simulink model "tank_flow"  (R2018b)
settings: Solver=ode1  StartTime=0.0  StopTime=170  FixedStep=.5  RelTol=1e-3  AbsTol=1e-6
PreLoadFcn:
  | sldemo_tankgui
StartFcn:
  | sldemo_tankgui start
StopFcn:
  | sldemo_tankgui stop
values from neighbouring files (symbols this model uses):
  Kp = 4/ts/b_lin    [tank_valve_PI_design.m]
undefined symbols (not defined in the file or in its folder): area, hilim, inflow, lolim, outflow
CloseFcn:
  | sldemo_tankgui done
Description:
  | Tank Fill and Empty with Animation
  | 
  | This example shows how to model the dynamics of liquid in a tank. The
  | associated animation provides a graphical display of the tank as it empties and
  | refills, based on user-defined tank parameters. The tank empties at the start
  | of the simulation and again part way through the simulation. When the simulation
  | is stopped, a plot is generated showing the liquid height and the states of the
  | two valves.
settings Model: ExtModeTrigMode=oneshot  ExtModeArmWhenConnect=off  ExtModeAutoUpdateStatusClock=off  Creator=The MathWorks, Inc.  LastModifiedBy=kjartan
settings SolverCC: AutoScaleAbsTol=off
settings DataIOCC: SaveFormat=Array  SignalLoggingName=sigsOut
settings OptimizationCC: InitFltsAndDblsToZero=on  LifeSpan=inf  BufferReusableBoundary=off
settings DebuggingCC: SaveWithParameterizedLinksMsg=none  UnderspecifiedInitializationDetection=Classic  MergeDetectMultiDrivingBlocksExec=none  SignalResolutionControl=TryResolveAllWithWarning  MultiTaskDSMMsg=warning  MultiTaskCondExecSysMsg=none  IntegerOverflowMsg=none  FcnCallInpInsideContextMsg=warning  BusObjectLabelMismatch=none  StateNameClashWarn=warning  SFUnexpectedBacktrackingDiag=warning  SFNoUnconditionalDefaultTransitionDiag=warning  SFExecutionAtInitializationDiag=none  IntegerSaturationMsg=none
settings HardwareCC: ProdBitPerPointer=32  ProdBitPerSizeT=32  ProdBitPerPtrDiffT=32  ProdLargestAtomicFloat=None  ProdIntDivRoundTo=Undefined  ProdEndianess=Unspecified  ProdWordSize=32  ProdHWDeviceType=32-bit Generic  TargetUnknown=on
settings ModelReferenceCC: PropagateSignalLabelsOutOfModel=off
settings SFSimCC: SimUseLocalCustomCode=off
settings RTWCC: Description=Generic Real-Time Target  RTWUseLocalCustomCode=off
settings CodeAppCC: StateflowObjectComments=on
settings GRTTargetCC: TargetFcnLib=ansi_tfl_tmw.mat  TargetLangStandard=C89/C90 (ANSI)  GeneratePreprocessorConditionals=Disable all  CombineOutputUpdateFcns=off  GRTInterface=on
settings ConfigComp: CovMetricSettings=dw  CovHtmlReporting=on  CovSaveCumulativeToWorkspaceVar=on  CovSaveSingleToWorkspaceVar=on  CovExternalEMLEnable=off

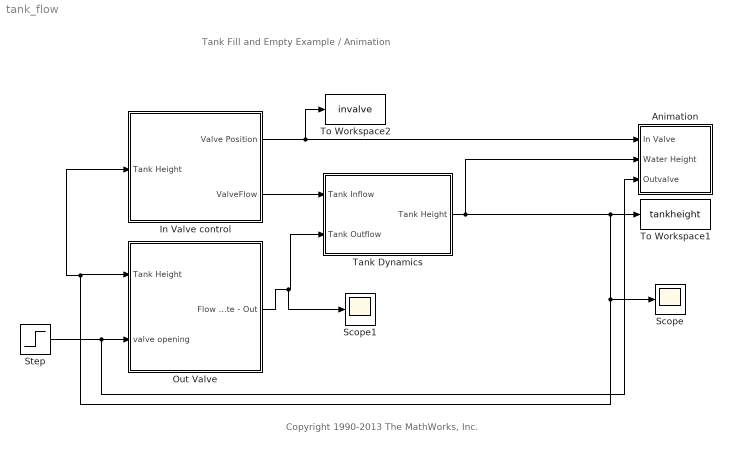
== system tank_flow ==
  note: Tank Fill and Empty Example / Animation
  note: Copyright 1990-2013 The MathWorks, Inc.
  Animation : Subsystem
      mask Display: disp('Animation\nControl')
  In Valve control : Subsystem  mask{hilim=hilim, inflow=inflow}
      mask prompts: hilim "Shut Off Height"; inflow "Flow Rate"
  Out Valve : Subsystem
  Scope : Scope
  Scope1 : Scope
  Step : Step  Time=3  SampleTime=0
  Tank Dynamics : Subsystem
  To Workspace1 : ToWorkspace  VariableName=tankheight  SampleTime=-1
  To Workspace2 : ToWorkspace  VariableName=invalve  SampleTime=-1
  wires:
  ? -> ?
  In Valve control/1(Valve Position) -> Animation/1(In Valve), To Workspace2/1
  Tank Dynamics/1(Tank Height) -> Animation/2(Water Height), Scope/1, In Valve control/1(Tank Height), Out Valve/1(Tank Height), To Workspace1/1
  In Valve control/2(ValveFlow) -> Tank Dynamics/1(Tank Inflow)
  Out Valve/1(Flow Rate - Out) -> Scope1/1, Tank Dynamics/2(Tank Outflow)
  Step/1 -> Animation/3(Outvalve), Out Valve/2(valve opening)

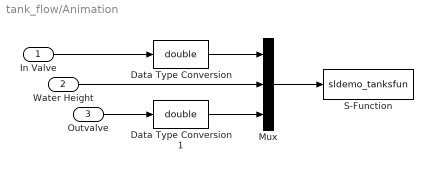
== system tank_flow/Animation ==
  In Valve : Inport
  Water Height : Inport  Port=2
  Outvalve : Inport  Port=3
  Data Type Conversion : DataTypeConversion  OutDataTypeStr=double  SaturateOnIntegerOverflow=on  RndMeth=Zero
  Data Type Conversion1 : DataTypeConversion  OutDataTypeStr=double  SaturateOnIntegerOverflow=on  RndMeth=Zero
  Mux : Mux  Inputs=3
  S-Function : S-Function  FunctionName=sldemo_tanksfun  Parameters=inflow,outflow,lolim,hilim,area  SFunctionDeploymentMode=off  EnableBusSupport=off
  wires:
  Outvalve/1 -> Data Type Conversion1/1
  Water Height/1 -> Mux/2
  Mux/1 -> S-Function/1
  In Valve/1 -> Data Type Conversion/1
  Data Type Conversion1/1 -> Mux/3
  Data Type Conversion/1 -> Mux/1

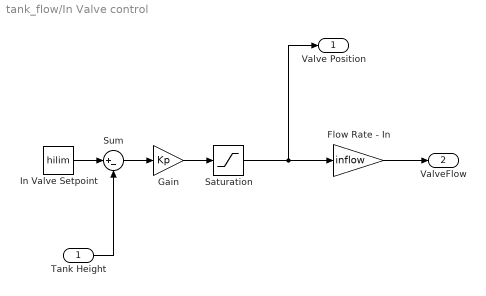
== system tank_flow/In Valve control ==
  Tank Height : Inport
  Flow Rate - In : Gain  Gain=inflow  OutDataTypeStr=Inherit: Inherit via back propagation  SaturateOnIntegerOverflow=on  ParamDataTypeStr=Inherit: Same as input
  Gain : Gain  Gain=Kp
  In Valve Setpoint : Constant  Value=hilim
  Saturation : Saturate  UpperLimit=1  LowerLimit=0
  Sum : Sum  Inputs=|+-
  Valve Position : Outport  InitialOutput=0
  ValveFlow : Outport  Port=2  InitialOutput=0
  wires:
  Flow Rate - In/1 -> ValveFlow/1
  Sum/1 -> Gain/1
  Tank Height/1 -> Sum/2
  In Valve Setpoint/1 -> Sum/1
  Saturation/1 -> Valve Position/1, Flow Rate - In/1
  Gain/1 -> Saturation/1

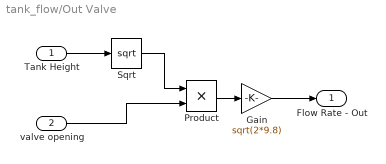
== system tank_flow/Out Valve ==
  Tank Height : Inport
  valve opening : Inport  Port=2
  Gain : Gain  Gain=sqrt(2*9.8)
  Product : Product
  Sqrt : Sqrt  SaturateOnIntegerOverflow=on
  Flow Rate - Out : Outport  InitialOutput=0
  wires:
  Tank Height/1 -> Sqrt/1
  Gain/1 -> Flow Rate - Out/1
  Sqrt/1 -> Product/1
  valve opening/1 -> Product/2
  Product/1 -> Gain/1

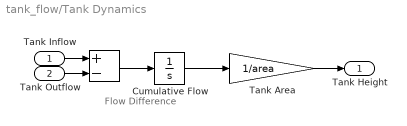
== system tank_flow/Tank Dynamics ==
  note: Flow
      | Difference
  Tank Inflow : Inport
  Tank Outflow : Inport  Port=2
  " " : Sum  Inputs=+-  SaturateOnIntegerOverflow=on  InputSameDT=on  OutDataTypeStr=Inherit: Same as first input
  Cumulative Flow : Integrator  InitialCondition=(hilim+lolim)/2*area
  Tank Area : Gain  Gain=1/area  SaturateOnIntegerOverflow=on  OutDataTypeStr=Inherit: Same as input  ParamDataTypeStr=Inherit: Same as input
  Tank Height : Outport  InitialOutput=0
  wires:
  Tank Outflow/1 -> " "/2
  Tank Inflow/1 -> " "/1
  " "/1 -> Cumulative Flow/1
  Cumulative Flow/1 -> Tank Area/1
  Tank Area/1 -> Tank Height/1
